simulink model "Model_3_1"  (R2021a)
settings: Solver=VariableStepAuto  StartTime=0.0  StopTime=10  RelTol=1e-3
InitFcn:
  | bx=0; %25
  | bl=0; %50
  | bc=0.01;
  | 
  | ml=2; %2
  | 
  | mc=0.5;
  | M2=0.5;
  | 
  | mt=5;
  | g=9.81;
  | l_ref=0.1;
  | l_ini=1;
  | l=l_ini;
  | x_ref=1; %5 3
  | n1=1; %5
  | n2=1;
  | 
  | L_2=0;  %chieu dai day nang ha
  | 
  | theta1_ini=0*pi/180;
  | theta2_ini=0*pi/180;  %2*pi/180
  | 
  | L_tai=0.2;
  | %ADRC' s parameter caculation
  | %b0 = (1)/(mc+mt+ml);
  | b0=(ml+mc)/(mt*mc+2*ml*mc+mt*ml+ml^2+mc^2); %Enhanced-coupling
  | %k_ESO = 100;
  | k_ESO = 100;
  | T_set  = 3; %5; 3
  | 
  | s_cl = -5.85/T_set;
  | Kp   = s_cl^2;
  | Kd   = -2*s_cl;
  | 
  | s_ESO = k_ESO*s_cl;
  | l1        = -3*s_ESO;
  | l2        = 3*( s_ESO)^2;
  | l3        = -(s_ESO)^3;
  | 
  | %b1 = (mt+mc)/(mc*ml +mc*mt+ml*mt);
  | b1=1/(ml+mc);
  | k_ESO1 =100; %100
  | T_set1  = 3;   %3
  | s_cl1 = -5.85/T_set1;
  | Kp1   = s_cl1^2;
  | Kd1   = -2*s_cl1;
  | 
  | s_ESO1 = k_ESO1*s_cl1;
  | l11        = -3*s_ESO1;
  | l21        = 3*( s_ESO1)^2;
  | l31        = -(s_ESO1)^3;
  | 
  | 
  | %L1=l_ini;
  | L11=0.55;
  | L2=0.1;
  | m1=2;
  | %m2=M2;
  | m=5;
  | ... (+39 lines)
libraries: neural x1137, simulink x36, simulink_extras x4
(part 6 of 45)

== system Model_3_1/26_12_theta1 bang 0 n1=5; n2=1 /Subsystem1/Fitness APS 1 ==
  e : Inport
  Abs : Abs
  Abs1 : Abs
  Integrator : Integrator
  MinMax Running Resettable : simulink/Math Operations/MinMax Running Resettable  Function=max  vinit=0.0
  Step : Step  Time=0.000001  Before=1  After=0  SampleTime=0
  IAE : Outport
  MAx : Outport  Port=2
  wires:
  Abs/1 -> Integrator/1
  Abs1/1 -> MinMax Running Resettable/1
  Step/1 -> MinMax Running Resettable/2
  e/1 -> Abs/1, Abs1/1
  Integrator/1 -> IAE/1
  MinMax Running Resettable/1 -> MAx/1

== system Model_3_1/26_12_theta1 bang 0 n1=5; n2=1 /Subsystem1/Fitness APS 2 ==
  e : Inport
  Abs : Abs
  Abs1 : Abs
  Integrator : Integrator
  MinMax Running Resettable : simulink/Math Operations/MinMax Running Resettable  Function=max  vinit=0.0
  Step : Step  Time=0.000001  Before=1  After=0  SampleTime=0
  IAE : Outport
  MAx : Outport  Port=2
  wires:
  Abs/1 -> Integrator/1
  Abs1/1 -> MinMax Running Resettable/1
  Step/1 -> MinMax Running Resettable/2
  e/1 -> Abs/1, Abs1/1
  Integrator/1 -> IAE/1
  MinMax Running Resettable/1 -> MAx/1

== system Model_3_1/26_12_theta1 bang 0 n1=5; n2=1 /Subsystem2/Fitness APS 1 ==
  e : Inport
  Abs : Abs
  Abs1 : Abs
  Integrator : Integrator
  MinMax Running Resettable : simulink/Math Operations/MinMax Running Resettable  Function=max  vinit=0.0
  Step : Step  Time=0.000001  Before=1  After=0  SampleTime=0
  IAE : Outport
  MAx : Outport  Port=2
  wires:
  Abs/1 -> Integrator/1
  Abs1/1 -> MinMax Running Resettable/1
  Step/1 -> MinMax Running Resettable/2
  e/1 -> Abs/1, Abs1/1
  Integrator/1 -> IAE/1
  MinMax Running Resettable/1 -> MAx/1

== system Model_3_1/26_12_theta1 bang 0 n1=5; n2=1 /Subsystem2/Fitness APS 2 ==
  e : Inport
  Abs : Abs
  Abs1 : Abs
  Integrator : Integrator
  MinMax Running Resettable : simulink/Math Operations/MinMax Running Resettable  Function=max  vinit=0.0
  Step : Step  Time=0.000001  Before=1  After=0  SampleTime=0
  IAE : Outport
  MAx : Outport  Port=2
  wires:
  Abs/1 -> Integrator/1
  Abs1/1 -> MinMax Running Resettable/1
  Step/1 -> MinMax Running Resettable/2
  e/1 -> Abs/1, Abs1/1
  Integrator/1 -> IAE/1
  MinMax Running Resettable/1 -> MAx/1

== system Model_3_1/26_12_theta1 bang 0 n1=5; n2=1 /Subsystem3/Fitness APS 1 ==
  e : Inport
  Abs : Abs
  Abs1 : Abs
  Integrator : Integrator
  MinMax Running Resettable : simulink/Math Operations/MinMax Running Resettable  Function=max  vinit=0.0
  Step : Step  Time=0.000001  Before=1  After=0  SampleTime=0
  IAE : Outport
  MAx : Outport  Port=2
  wires:
  Abs/1 -> Integrator/1
  Abs1/1 -> MinMax Running Resettable/1
  Step/1 -> MinMax Running Resettable/2
  e/1 -> Abs/1, Abs1/1
  Integrator/1 -> IAE/1
  MinMax Running Resettable/1 -> MAx/1

== system Model_3_1/26_12_theta1 bang 0 n1=5; n2=1 /Subsystem3/Fitness APS 2 ==
  e : Inport
  Abs : Abs
  Abs1 : Abs
  Integrator : Integrator
  MinMax Running Resettable : simulink/Math Operations/MinMax Running Resettable  Function=max  vinit=0.0
  Step : Step  Time=0.000001  Before=1  After=0  SampleTime=0
  IAE : Outport
  MAx : Outport  Port=2
  wires:
  Abs/1 -> Integrator/1
  Abs1/1 -> MinMax Running Resettable/1
  Step/1 -> MinMax Running Resettable/2
  e/1 -> Abs/1, Abs1/1
  Integrator/1 -> IAE/1
  MinMax Running Resettable/1 -> MAx/1

== system Model_3_1/26_12_theta1 bang 0 n1=5; n2=1 /Subsystem4/Fitness APS 1 ==
  e : Inport
  Abs : Abs
  Abs1 : Abs
  Integrator : Integrator
  MinMax Running Resettable : simulink/Math Operations/MinMax Running Resettable  Function=max  vinit=0.0
  Step : Step  Time=0.000001  Before=1  After=0  SampleTime=0
  IAE : Outport
  MAx : Outport  Port=2
  wires:
  Abs/1 -> Integrator/1
  Abs1/1 -> MinMax Running Resettable/1
  Step/1 -> MinMax Running Resettable/2
  e/1 -> Abs/1, Abs1/1
  Integrator/1 -> IAE/1
  MinMax Running Resettable/1 -> MAx/1

== system Model_3_1/26_12_theta1 bang 0 n1=5; n2=1 /Subsystem4/Fitness APS 2 ==
  e : Inport
  Abs : Abs
  Abs1 : Abs
  Integrator : Integrator
  MinMax Running Resettable : simulink/Math Operations/MinMax Running Resettable  Function=max  vinit=0.0
  Step : Step  Time=0.000001  Before=1  After=0  SampleTime=0
  IAE : Outport
  MAx : Outport  Port=2
  wires:
  Abs/1 -> Integrator/1
  Abs1/1 -> MinMax Running Resettable/1
  Step/1 -> MinMax Running Resettable/2
  e/1 -> Abs/1, Abs1/1
  Integrator/1 -> IAE/1
  MinMax Running Resettable/1 -> MAx/1

== system Model_3_1/26_12_theta1 bang 0 n1=5; n2=1 /Subsystem5/Fitness APS 1 ==
  e : Inport
  Abs : Abs
  Abs1 : Abs
  Integrator : Integrator
  MinMax Running Resettable : simulink/Math Operations/MinMax Running Resettable  Function=max  vinit=0.0
  Step : Step  Time=0.000001  Before=1  After=0  SampleTime=0
  IAE : Outport
  MAx : Outport  Port=2
  wires:
  Abs/1 -> Integrator/1
  Abs1/1 -> MinMax Running Resettable/1
  Step/1 -> MinMax Running Resettable/2
  e/1 -> Abs/1, Abs1/1
  Integrator/1 -> IAE/1
  MinMax Running Resettable/1 -> MAx/1

== system Model_3_1/26_12_theta1 bang 0 n1=5; n2=1 /Subsystem5/Fitness APS 2 ==
  e : Inport
  Abs : Abs
  Abs1 : Abs
  Integrator : Integrator
  MinMax Running Resettable : simulink/Math Operations/MinMax Running Resettable  Function=max  vinit=0.0
  Step : Step  Time=0.000001  Before=1  After=0  SampleTime=0
  IAE : Outport
  MAx : Outport  Port=2
  wires:
  Abs/1 -> Integrator/1
  Abs1/1 -> MinMax Running Resettable/1
  Step/1 -> MinMax Running Resettable/2
  e/1 -> Abs/1, Abs1/1
  Integrator/1 -> IAE/1
  MinMax Running Resettable/1 -> MAx/1

== system Model_3_1/26_12_theta1 bang 0 n1=5; n2=1 /Subsystem6/Fitness APS 1 ==
  e : Inport
  Abs : Abs
  Abs1 : Abs
  Integrator : Integrator
  MinMax Running Resettable : simulink/Math Operations/MinMax Running Resettable  Function=max  vinit=0.0
  Step : Step  Time=0.000001  Before=1  After=0  SampleTime=0
  IAE : Outport
  MAx : Outport  Port=2
  wires:
  Abs/1 -> Integrator/1
  Abs1/1 -> MinMax Running Resettable/1
  Step/1 -> MinMax Running Resettable/2
  e/1 -> Abs/1, Abs1/1
  Integrator/1 -> IAE/1
  MinMax Running Resettable/1 -> MAx/1

== system Model_3_1/26_12_theta1 bang 0 n1=5; n2=1 /Subsystem6/Fitness APS 2 ==
  e : Inport
  Abs : Abs
  Abs1 : Abs
  Integrator : Integrator
  MinMax Running Resettable : simulink/Math Operations/MinMax Running Resettable  Function=max  vinit=0.0
  Step : Step  Time=0.000001  Before=1  After=0  SampleTime=0
  IAE : Outport
  MAx : Outport  Port=2
  wires:
  Abs/1 -> Integrator/1
  Abs1/1 -> MinMax Running Resettable/1
  Step/1 -> MinMax Running Resettable/2
  e/1 -> Abs/1, Abs1/1
  Integrator/1 -> IAE/1
  MinMax Running Resettable/1 -> MAx/1

== system Model_3_1/26_12_theta1 bang 0 n1=5; n2=1 /ko co FL_25.12_2/Layer 1 ==
  "p{1}" : Inport  PortDimensions=2
      mask Display: e = 0.06;c1 = [120 230 180]/255;c2 = ([120 230 180]+0)/(256+128);c3 = ([120 230 180]+128)/(256+128);patch([0 1 1 0],[0 0 1 1],c1);patch([0 1 1 1-e 1-e 0+e],[0 0 1 1-e 0+e 0+e],c2);patch([0 0 1 1-e 0+e 0+e],[0 1 1 1-e 1-e 0+e],c3);plot([0 1 1 0 0],[0 0 1 1 0]);
  Delays 1 : Subsystem
      mask Display: e = 0.06;c1 = [120 150 230]/255;c2 = ([120 150 230]+0)/383;c3 = ([120 150 230]+128)/383;patch([0 1 1 0],[0 0 1 1],c1);patch([0 1 1 1-e 1-e 0+e],[0 0 1 1-e 0+e 0+e],c2);patch([0 0 1 1-e 0+e 0+e],[0 1 1 1-e 1-e 0+e],c3);plot([0 1 1 0 0],[0 0 1 1 0]);disp('0');
  "IW{1,1}" : Subsystem
      mask Display: e = 0.06;c1 = [120 150 230]/255;c2 = ([120 150 230]+0)/383;c3 = ([120 150 230]+128)/383;patch([0 1 1 0],[0 0 1 1],c1);patch([0 1 1 1-e 1-e 0+e],[0 0 1 1-e 0+e 0+e],c2);patch([0 0 1 1-e 0+e 0+e],[0 1 1 1-e 1-e 0+e],c3);plot([0 1 1 0 0],[0 0 1 1 0]);disp('W');
  "b{1}" : Constant  Value=[0.83255461115769768820626950400765053927898406982421875;0.83255461115769768820626950400765053927898406982421875;0.83255461115769768820626950400765053927898406982421875;0.83255461115769768820626950400765053927898406982421875;0.83255461115769768820626950400765053927898406982421875;0.83255461115769768820626950400765053927898406982421875;0.83255461115769768820626950400765053927898406982421875;0.83255461115769768820626950400765053927898406982421875;0.83255461115769768820626950400765053927898406982421875;0.83255461115769768820626950400765053927898406982421875;0.83255461115769768820626950400765053927898406982421875;0.83255461115769768820626950400765053927898406982421875;0.83255461115769768820626950400765053927898406982421875;0.83255461115769768820626950400765053927898406982421875;0.83255461115769768820626950400765053927898406982421875;0.83255461115769768820626950400765053927898406982421875;0.83255461115769768820626950400765053927898406982421875;0.83255461115769768820626950400765053927898406982421875;0.83255461115769768820626950400765053927898406982421875;0.83255461115769768820626950400765053927898406982421875;0.83255461115769768820626950400765053927898406982421875;0.83255461115769768820626950400765053927898406982421875;0.83255461115769768820626950400765053927898406982421875;0.83255461115769768820626950400765053927898406982421875;0.83255461115769768820626950400765053927898406982421875;0.83255461115769768820626950400765053927898406982421875;0.83255461115769768820626950400765053927898406982421875;0.83255461115769768820626950400765053927898406982421875;0.83255461115769768820626950400765053927898406982421875;0.83255461115769768820626950400765053927898406982421875;0.83255461115769768820626950400765053927898406982421875;0.83255461115769768820626950400765053927898406982421875;0.83255461115769768820626950400765053927898406982421875;0.83255461115769768820626950400765053927898406982421875;0.83255461115769768820626950400765053927898406982421875;0.83255461115769768820626950400765053927898406982421875;0.83255461115769768820626950400765053927898406982421875;0.83255461115769768820626950400765053927898406982421875;0.83255461115769768820626950400765053927898406982421875;0.83255461115769768820626950400765053927898406982421875;0.83255461115769768820626950400765053927898406982421875;0.83255461115769768820626950400765053927898406982421875;0.83255461115769768820626950400765053927898406982421875;0.83255461115769768820626950400765053927898406982421875;0.83255461115769768820626950400765053927898406982421875;0.83255461115769768820626950400765053927898406982421875]
      mask Display: e = 0.06;c1 = [120 150 230]/255;c2 = ([120 150 230]+0)/383;c3 = ([120 150 230]+128)/383;patch([0 1 1 0],[0 0 1 1],c1);patch([0 1 1 1-e 1-e 0+e],[0 0 1 1-e 0+e 0+e],c2);patch([0 0 1 1-e 0+e 0+e],[0 1 1 1-e 1-e 0+e],c3);plot([0 1 1 0 0],[0 0 1 1 0]);disp('b');
  netprod : Product  InputSameDT=on  RndMeth=Zero  SaturateOnIntegerOverflow=on  OutDataTypeStr=Inherit: Same as first input
      mask Display: e = 0.06;c1 = [120 150 230]/255;c2 = ([120 150 230]+0)/383;c3 = ([120 150 230]+128)/383;patch([0 1 1 0],[0 0 1 1],c1);patch([0 1 1 1-e 1-e 0+e],[0 0 1 1-e 0+e 0+e],c2);patch([0 0 1 1-e 0+e 0+e],[0 1 1 1-e 1-e 0+e],c3);plot([0 1 1 0 0],[0 0 1 1 0]);disp('*');
  radbas : neural/Transfer Functions/radbas
      settings: SourceProductBaseCode=NN
  "a{1}" : Outport  InitialOutput=[0;0;0;0;0;0;0;0;0;0;0;0;0;0;0;0;0;0;0;0;0;0;0;0;0;0;0;0;0;0;0;0;0;0;0;0;0;0;0;0;0;0;0;0;0;0]
      mask Display: e = 0.06;c1 = [120 230 180]/255;c2 = ([120 230 180]+0)/(256+128);c3 = ([120 230 180]+128)/(256+128);patch([0 1 1 0],[0 0 1 1],c1);patch([0 1 1 1-e 1-e 0+e],[0 0 1 1-e 0+e 0+e],c2);patch([0 0 1 1-e 0+e 0+e],[0 1 1 1-e 1-e 0+e],c3);plot([0 1 1 0 0],[0 0 1 1 0]);
  wires:
  "p{1}"/1 -> Delays 1/1("p{1}")
  Delays 1/1("pd{1,1}") -> "IW{1,1}"/1("pd{1,1}")
  "IW{1,1}"/1("iz{1,1}") -> netprod/1
  "b{1}"/1 -> netprod/2
  netprod/1 -> radbas/1
  radbas/1 -> "a{1}"/1

== system Model_3_1/26_12_theta1 bang 0 n1=5; n2=1 /ko co FL_25.12_2/Layer 2 ==
  "a{1} " : Inport  PortDimensions=46
      mask Display: e = 0.06;c1 = [120 230 180]/255;c2 = ([120 230 180]+0)/(256+128);c3 = ([120 230 180]+128)/(256+128);patch([0 1 1 0],[0 0 1 1],c1);patch([0 1 1 1-e 1-e 0+e],[0 0 1 1-e 0+e 0+e],c2);patch([0 0 1 1-e 0+e 0+e],[0 1 1 1-e 1-e 0+e],c3);plot([0 1 1 0 0],[0 0 1 1 0]);
  Delays 1 : Subsystem
      mask Display: e = 0.06;c1 = [120 150 230]/255;c2 = ([120 150 230]+0)/383;c3 = ([120 150 230]+128)/383;patch([0 1 1 0],[0 0 1 1],c1);patch([0 1 1 1-e 1-e 0+e],[0 0 1 1-e 0+e 0+e],c2);patch([0 0 1 1-e 0+e 0+e],[0 1 1 1-e 1-e 0+e],c3);plot([0 1 1 0 0],[0 0 1 1 0]);disp('0');
  "LW{2,1}" : Subsystem
      mask Display: e = 0.06;c1 = [120 150 230]/255;c2 = ([120 150 230]+0)/383;c3 = ([120 150 230]+128)/383;patch([0 1 1 0],[0 0 1 1],c1);patch([0 1 1 1-e 1-e 0+e],[0 0 1 1-e 0+e 0+e],c2);patch([0 0 1 1-e 0+e 0+e],[0 1 1 1-e 1-e 0+e],c3);plot([0 1 1 0 0],[0 0 1 1 0]);disp('W');
  "b{2}" : Constant  Value=[-128346.528805981113691814243793487548828125;1328.286650372559279276174493134021759033203125;-25277.92810932771317311562597751617431640625]
      mask Display: e = 0.06;c1 = [120 150 230]/255;c2 = ([120 150 230]+0)/383;c3 = ([120 150 230]+128)/383;patch([0 1 1 0],[0 0 1 1],c1);patch([0 1 1 1-e 1-e 0+e],[0 0 1 1-e 0+e 0+e],c2);patch([0 0 1 1-e 0+e 0+e],[0 1 1 1-e 1-e 0+e],c3);plot([0 1 1 0 0],[0 0 1 1 0]);disp('b');
  netsum : Sum  Inputs=2  InputSameDT=on  SaturateOnIntegerOverflow=on  OutDataTypeStr=Inherit: Same as first input
      mask Display: e = 0.06;c1 = [120 150 230]/255;c2 = ([120 150 230]+0)/383;c3 = ([120 150 230]+128)/383;patch([0 1 1 0],[0 0 1 1],c1);patch([0 1 1 1-e 1-e 0+e],[0 0 1 1-e 0+e 0+e],c2);patch([0 0 1 1-e 0+e 0+e],[0 1 1 1-e 1-e 0+e],c3);plot([0 1 1 0 0],[0 0 1 1 0]);disp('+');
  purelin : neural/Transfer Functions/purelin
  "a{2}" : Outport  InitialOutput=[0;0;0]
      mask Display: e = 0.06;c1 = [120 230 180]/255;c2 = ([120 230 180]+0)/(256+128);c3 = ([120 230 180]+128)/(256+128);patch([0 1 1 0],[0 0 1 1],c1);patch([0 1 1 1-e 1-e 0+e],[0 0 1 1-e 0+e 0+e],c2);patch([0 0 1 1-e 0+e 0+e],[0 1 1 1-e 1-e 0+e],c3);plot([0 1 1 0 0],[0 0 1 1 0]);
  wires:
  "a{1} "/1 -> Delays 1/1("p{2}")
  Delays 1/1("pd{2,1}") -> "LW{2,1}"/1("ad{2,1}")
  "LW{2,1}"/1("lz{2,1}") -> netsum/1
  "b{2}"/1 -> netsum/2
  netsum/1 -> purelin/1
  purelin/1 -> "a{2}"/1

== system Model_3_1/26_12_theta1 bang 0 n1=5; n2=1 /ko co FL_25.12_2/Process Input 1 ==
  x : Inport  PortDimensions=2
      mask Display: e = 0.06;c1 = [120 230 180]/255;c2 = ([120 230 180]+0)/(256+128);c3 = ([120 230 180]+128)/(256+128);patch([0 1 1 0],[0 0 1 1],c1);patch([0 1 1 1-e 1-e 0+e],[0 0 1 1-e 0+e 0+e],c2);patch([0 0 1 1-e 0+e 0+e],[0 1 1 1-e 1-e 0+e],c3);plot([0 1 1 0 0],[0 0 1 1 0]);
  p : Outport  PortDimensions=2
      mask Display: e = 0.06;c1 = [120 230 180]/255;c2 = ([120 230 180]+0)/(256+128);c3 = ([120 230 180]+128)/(256+128);patch([0 1 1 0],[0 0 1 1],c1);patch([0 1 1 1-e 1-e 0+e],[0 0 1 1-e 0+e 0+e],c2);patch([0 0 1 1-e 0+e 0+e],[0 1 1 1-e 1-e 0+e],c3);plot([0 1 1 0 0],[0 0 1 1 0]);
  wires:
  x/1 -> p/1

== system Model_3_1/26_12_theta1 bang 0 n1=5; n2=1 /ko co FL_25.12_2/Process Output 1 ==
  a : Inport  PortDimensions=3
      mask Display: e = 0.06;c1 = [120 230 180]/255;c2 = ([120 230 180]+0)/(256+128);c3 = ([120 230 180]+128)/(256+128);patch([0 1 1 0],[0 0 1 1],c1);patch([0 1 1 1-e 1-e 0+e],[0 0 1 1-e 0+e 0+e],c2);patch([0 0 1 1-e 0+e 0+e],[0 1 1 1-e 1-e 0+e],c3);plot([0 1 1 0 0],[0 0 1 1 0]);
  y : Outport  PortDimensions=3
      mask Display: e = 0.06;c1 = [120 230 180]/255;c2 = ([120 230 180]+0)/(256+128);c3 = ([120 230 180]+128)/(256+128);patch([0 1 1 0],[0 0 1 1],c1);patch([0 1 1 1-e 1-e 0+e],[0 0 1 1-e 0+e 0+e],c2);patch([0 0 1 1-e 0+e 0+e],[0 1 1 1-e 1-e 0+e],c3);plot([0 1 1 0 0],[0 0 1 1 0]);
  wires:
  a/1 -> y/1

== system Model_3_1/26_12_theta1 bang 0 n1=5; n2=1 /ko co FL_26.1_1/Layer 1 ==
  "p{1}" : Inport  PortDimensions=2
      mask Display: e = 0.06;c1 = [120 230 180]/255;c2 = ([120 230 180]+0)/(256+128);c3 = ([120 230 180]+128)/(256+128);patch([0 1 1 0],[0 0 1 1],c1);patch([0 1 1 1-e 1-e 0+e],[0 0 1 1-e 0+e 0+e],c2);patch([0 0 1 1-e 0+e 0+e],[0 1 1 1-e 1-e 0+e],c3);plot([0 1 1 0 0],[0 0 1 1 0]);
  Delays 1 : Subsystem
      mask Display: e = 0.06;c1 = [120 150 230]/255;c2 = ([120 150 230]+0)/383;c3 = ([120 150 230]+128)/383;patch([0 1 1 0],[0 0 1 1],c1);patch([0 1 1 1-e 1-e 0+e],[0 0 1 1-e 0+e 0+e],c2);patch([0 0 1 1-e 0+e 0+e],[0 1 1 1-e 1-e 0+e],c3);plot([0 1 1 0 0],[0 0 1 1 0]);disp('0');
  "IW{1,1}" : Subsystem
      mask Display: e = 0.06;c1 = [120 150 230]/255;c2 = ([120 150 230]+0)/383;c3 = ([120 150 230]+128)/383;patch([0 1 1 0],[0 0 1 1],c1);patch([0 1 1 1-e 1-e 0+e],[0 0 1 1-e 0+e 0+e],c2);patch([0 0 1 1-e 0+e 0+e],[0 1 1 1-e 1-e 0+e],c3);plot([0 1 1 0 0],[0 0 1 1 0]);disp('W');
  "b{1}" : Constant  Value=[0.83255461115769768820626950400765053927898406982421875;0.83255461115769768820626950400765053927898406982421875;0.83255461115769768820626950400765053927898406982421875;0.83255461115769768820626950400765053927898406982421875;0.83255461115769768820626950400765053927898406982421875;0.83255461115769768820626950400765053927898406982421875;0.83255461115769768820626950400765053927898406982421875;0.83255461115769768820626950400765053927898406982421875;0.83255461115769768820626950400765053927898406982421875;0.83255461115769768820626950400765053927898406982421875;0.83255461115769768820626950400765053927898406982421875;0.83255461115769768820626950400765053927898406982421875;0.83255461115769768820626950400765053927898406982421875;0.83255461115769768820626950400765053927898406982421875;0.83255461115769768820626950400765053927898406982421875;0.83255461115769768820626950400765053927898406982421875;0.83255461115769768820626950400765053927898406982421875;0.83255461115769768820626950400765053927898406982421875;0.83255461115769768820626950400765053927898406982421875;0.83255461115769768820626950400765053927898406982421875;0.83255461115769768820626950400765053927898406982421875;0.83255461115769768820626950400765053927898406982421875;0.83255461115769768820626950400765053927898406982421875;0.83255461115769768820626950400765053927898406982421875;0.83255461115769768820626950400765053927898406982421875;0.83255461115769768820626950400765053927898406982421875;0.83255461115769768820626950400765053927898406982421875;0.83255461115769768820626950400765053927898406982421875;0.83255461115769768820626950400765053927898406982421875;0.83255461115769768820626950400765053927898406982421875;0.83255461115769768820626950400765053927898406982421875;0.83255461115769768820626950400765053927898406982421875;0.83255461115769768820626950400765053927898406982421875;0.83255461115769768820626950400765053927898406982421875;0.83255461115769768820626950400765053927898406982421875;0.83255461115769768820626950400765053927898406982421875;0.83255461115769768820626950400765053927898406982421875;0.83255461115769768820626950400765053927898406982421875;0.83255461115769768820626950400765053927898406982421875;0.83255461115769768820626950400765053927898406982421875;0.83255461115769768820626950400765053927898406982421875;0.83255461115769768820626950400765053927898406982421875;0.83255461115769768820626950400765053927898406982421875;0.83255461115769768820626950400765053927898406982421875;0.83255461115769768820626950400765053927898406982421875;0.83255461115769768820626950400765053927898406982421875]
      mask Display: e = 0.06;c1 = [120 150 230]/255;c2 = ([120 150 230]+0)/383;c3 = ([120 150 230]+128)/383;patch([0 1 1 0],[0 0 1 1],c1);patch([0 1 1 1-e 1-e 0+e],[0 0 1 1-e 0+e 0+e],c2);patch([0 0 1 1-e 0+e 0+e],[0 1 1 1-e 1-e 0+e],c3);plot([0 1 1 0 0],[0 0 1 1 0]);disp('b');
  netprod : Product  InputSameDT=on  RndMeth=Zero  SaturateOnIntegerOverflow=on  OutDataTypeStr=Inherit: Same as first input
      mask Display: e = 0.06;c1 = [120 150 230]/255;c2 = ([120 150 230]+0)/383;c3 = ([120 150 230]+128)/383;patch([0 1 1 0],[0 0 1 1],c1);patch([0 1 1 1-e 1-e 0+e],[0 0 1 1-e 0+e 0+e],c2);patch([0 0 1 1-e 0+e 0+e],[0 1 1 1-e 1-e 0+e],c3);plot([0 1 1 0 0],[0 0 1 1 0]);disp('*');
  radbas : neural/Transfer Functions/radbas
      settings: SourceProductBaseCode=NN
  "a{1}" : Outport  InitialOutput=[0;0;0;0;0;0;0;0;0;0;0;0;0;0;0;0;0;0;0;0;0;0;0;0;0;0;0;0;0;0;0;0;0;0;0;0;0;0;0;0;0;0;0;0;0;0]
      mask Display: e = 0.06;c1 = [120 230 180]/255;c2 = ([120 230 180]+0)/(256+128);c3 = ([120 230 180]+128)/(256+128);patch([0 1 1 0],[0 0 1 1],c1);patch([0 1 1 1-e 1-e 0+e],[0 0 1 1-e 0+e 0+e],c2);patch([0 0 1 1-e 0+e 0+e],[0 1 1 1-e 1-e 0+e],c3);plot([0 1 1 0 0],[0 0 1 1 0]);
  wires:
  "p{1}"/1 -> Delays 1/1("p{1}")
  Delays 1/1("pd{1,1}") -> "IW{1,1}"/1("pd{1,1}")
  "IW{1,1}"/1("iz{1,1}") -> netprod/1
  "b{1}"/1 -> netprod/2
  netprod/1 -> radbas/1
  radbas/1 -> "a{1}"/1

== system Model_3_1/26_12_theta1 bang 0 n1=5; n2=1 /ko co FL_26.1_1/Layer 2 ==
  "a{1} " : Inport  PortDimensions=46
      mask Display: e = 0.06;c1 = [120 230 180]/255;c2 = ([120 230 180]+0)/(256+128);c3 = ([120 230 180]+128)/(256+128);patch([0 1 1 0],[0 0 1 1],c1);patch([0 1 1 1-e 1-e 0+e],[0 0 1 1-e 0+e 0+e],c2);patch([0 0 1 1-e 0+e 0+e],[0 1 1 1-e 1-e 0+e],c3);plot([0 1 1 0 0],[0 0 1 1 0]);
  Delays 1 : Subsystem
      mask Display: e = 0.06;c1 = [120 150 230]/255;c2 = ([120 150 230]+0)/383;c3 = ([120 150 230]+128)/383;patch([0 1 1 0],[0 0 1 1],c1);patch([0 1 1 1-e 1-e 0+e],[0 0 1 1-e 0+e 0+e],c2);patch([0 0 1 1-e 0+e 0+e],[0 1 1 1-e 1-e 0+e],c3);plot([0 1 1 0 0],[0 0 1 1 0]);disp('0');
  "LW{2,1}" : Subsystem
      mask Display: e = 0.06;c1 = [120 150 230]/255;c2 = ([120 150 230]+0)/383;c3 = ([120 150 230]+128)/383;patch([0 1 1 0],[0 0 1 1],c1);patch([0 1 1 1-e 1-e 0+e],[0 0 1 1-e 0+e 0+e],c2);patch([0 0 1 1-e 0+e 0+e],[0 1 1 1-e 1-e 0+e],c3);plot([0 1 1 0 0],[0 0 1 1 0]);disp('W');
  "b{2}" : Constant  Value=[-121700.422889903260511346161365509033203125;2285.68691207953406774322502315044403076171875;-58069.0026805897723534144461154937744140625]
      mask Display: e = 0.06;c1 = [120 150 230]/255;c2 = ([120 150 230]+0)/383;c3 = ([120 150 230]+128)/383;patch([0 1 1 0],[0 0 1 1],c1);patch([0 1 1 1-e 1-e 0+e],[0 0 1 1-e 0+e 0+e],c2);patch([0 0 1 1-e 0+e 0+e],[0 1 1 1-e 1-e 0+e],c3);plot([0 1 1 0 0],[0 0 1 1 0]);disp('b');
  netsum : Sum  Inputs=2  InputSameDT=on  SaturateOnIntegerOverflow=on  OutDataTypeStr=Inherit: Same as first input
      mask Display: e = 0.06;c1 = [120 150 230]/255;c2 = ([120 150 230]+0)/383;c3 = ([120 150 230]+128)/383;patch([0 1 1 0],[0 0 1 1],c1);patch([0 1 1 1-e 1-e 0+e],[0 0 1 1-e 0+e 0+e],c2);patch([0 0 1 1-e 0+e 0+e],[0 1 1 1-e 1-e 0+e],c3);plot([0 1 1 0 0],[0 0 1 1 0]);disp('+');
  purelin : neural/Transfer Functions/purelin
  "a{2}" : Outport  InitialOutput=[0;0;0]
      mask Display: e = 0.06;c1 = [120 230 180]/255;c2 = ([120 230 180]+0)/(256+128);c3 = ([120 230 180]+128)/(256+128);patch([0 1 1 0],[0 0 1 1],c1);patch([0 1 1 1-e 1-e 0+e],[0 0 1 1-e 0+e 0+e],c2);patch([0 0 1 1-e 0+e 0+e],[0 1 1 1-e 1-e 0+e],c3);plot([0 1 1 0 0],[0 0 1 1 0]);
  wires:
  "a{1} "/1 -> Delays 1/1("p{2}")
  Delays 1/1("pd{2,1}") -> "LW{2,1}"/1("ad{2,1}")
  "LW{2,1}"/1("lz{2,1}") -> netsum/1
  "b{2}"/1 -> netsum/2
  netsum/1 -> purelin/1
  purelin/1 -> "a{2}"/1

== system Model_3_1/26_12_theta1 bang 0 n1=5; n2=1 /ko co FL_26.1_1/Process Input 1 ==
  x : Inport  PortDimensions=2
      mask Display: e = 0.06;c1 = [120 230 180]/255;c2 = ([120 230 180]+0)/(256+128);c3 = ([120 230 180]+128)/(256+128);patch([0 1 1 0],[0 0 1 1],c1);patch([0 1 1 1-e 1-e 0+e],[0 0 1 1-e 0+e 0+e],c2);patch([0 0 1 1-e 0+e 0+e],[0 1 1 1-e 1-e 0+e],c3);plot([0 1 1 0 0],[0 0 1 1 0]);
  p : Outport  PortDimensions=2
      mask Display: e = 0.06;c1 = [120 230 180]/255;c2 = ([120 230 180]+0)/(256+128);c3 = ([120 230 180]+128)/(256+128);patch([0 1 1 0],[0 0 1 1],c1);patch([0 1 1 1-e 1-e 0+e],[0 0 1 1-e 0+e 0+e],c2);patch([0 0 1 1-e 0+e 0+e],[0 1 1 1-e 1-e 0+e],c3);plot([0 1 1 0 0],[0 0 1 1 0]);
  wires:
  x/1 -> p/1

== system Model_3_1/26_12_theta1 bang 0 n1=5; n2=1 /ko co FL_26.1_1/Process Output 1 ==
  a : Inport  PortDimensions=3
      mask Display: e = 0.06;c1 = [120 230 180]/255;c2 = ([120 230 180]+0)/(256+128);c3 = ([120 230 180]+128)/(256+128);patch([0 1 1 0],[0 0 1 1],c1);patch([0 1 1 1-e 1-e 0+e],[0 0 1 1-e 0+e 0+e],c2);patch([0 0 1 1-e 0+e 0+e],[0 1 1 1-e 1-e 0+e],c3);plot([0 1 1 0 0],[0 0 1 1 0]);
  y : Outport  PortDimensions=3
      mask Display: e = 0.06;c1 = [120 230 180]/255;c2 = ([120 230 180]+0)/(256+128);c3 = ([120 230 180]+128)/(256+128);patch([0 1 1 0],[0 0 1 1],c1);patch([0 1 1 1-e 1-e 0+e],[0 0 1 1-e 0+e 0+e],c2);patch([0 0 1 1-e 0+e 0+e],[0 1 1 1-e 1-e 0+e],c3);plot([0 1 1 0 0],[0 0 1 1 0]);
  wires:
  a/1 -> y/1

== system Model_3_1/3_1_theta1 bang 0 n1=1; n2=1 2/ETM1/ETM1 ==
  In1 : Inport
  Gain : Gain  Gain=A1_etm4_1
  Gain1 : Gain  Gain=A2_etm4_1
  Gain2 : Gain  Gain=A3_etm4_1
  Gain3 : Gain  Gain=A4_etm4_1
  Sum : Sum  Inputs=++++
  Transport Delay : TransportDelay  DelayTime=t1_etm4_1
  Transport Delay1 : TransportDelay  DelayTime=t2_etm4_1
  Transport Delay2 : TransportDelay  DelayTime=t3_etm4_1
  Out1 : Outport
  wires:
  In1/1 -> Gain1/1, Gain3/1, Gain2/1, Gain/1
  Gain1/1 -> Transport Delay/1
  Transport Delay/1 -> Sum/2
  Sum/1 -> Out1/1
  Gain2/1 -> Transport Delay1/1
  Gain/1 -> Sum/1
  Transport Delay1/1 -> Sum/3
  Gain3/1 -> Transport Delay2/1
  Transport Delay2/1 -> Sum/4

== system Model_3_1/3_1_theta1 bang 0 n1=1; n2=1 2/ETM1/ETM4 ==
  In1 : Inport
  Gain : Gain  Gain=A1_etm4_2
  Gain1 : Gain  Gain=A2_etm4_2
  Gain2 : Gain  Gain=A3_etm4_2
  Gain3 : Gain  Gain=A4_etm4_2
  Sum : Sum  Inputs=++++
  Transport Delay : TransportDelay  DelayTime=t1_etm4_2
  Transport Delay1 : TransportDelay  DelayTime=t2_etm4_2
  Transport Delay2 : TransportDelay  DelayTime=t3_etm4_2
  Out1 : Outport
  wires:
  In1/1 -> Gain1/1, Gain3/1, Gain2/1, Gain/1
  Gain1/1 -> Transport Delay/1
  Transport Delay/1 -> Sum/2
  Sum/1 -> Out1/1
  Gain2/1 -> Transport Delay1/1
  Gain/1 -> Sum/1
  Transport Delay1/1 -> Sum/3
  Gain3/1 -> Transport Delay2/1
  Transport Delay2/1 -> Sum/4

== system Model_3_1/3_1_theta1 bang 0 n1=1; n2=1 2/ETM2/ETM1 ==
  In1 : Inport
  Gain : Gain  Gain=A1_etm4_1
  Gain1 : Gain  Gain=A2_etm4_1
  Gain2 : Gain  Gain=A3_etm4_1
  Gain3 : Gain  Gain=A4_etm4_1
  Sum : Sum  Inputs=++++
  Transport Delay : TransportDelay  DelayTime=t1_etm4_1
  Transport Delay1 : TransportDelay  DelayTime=t2_etm4_1
  Transport Delay2 : TransportDelay  DelayTime=t3_etm4_1
  Out1 : Outport
  wires:
  In1/1 -> Gain1/1, Gain3/1, Gain2/1, Gain/1
  Gain1/1 -> Transport Delay/1
  Transport Delay/1 -> Sum/2
  Sum/1 -> Out1/1
  Gain2/1 -> Transport Delay1/1
  Gain/1 -> Sum/1
  Transport Delay1/1 -> Sum/3
  Gain3/1 -> Transport Delay2/1
  Transport Delay2/1 -> Sum/4

== system Model_3_1/3_1_theta1 bang 0 n1=1; n2=1 2/ETM2/ETM4 ==
  In1 : Inport
  Gain : Gain  Gain=A1_etm4_2
  Gain1 : Gain  Gain=A2_etm4_2
  Gain2 : Gain  Gain=A3_etm4_2
  Gain3 : Gain  Gain=A4_etm4_2
  Sum : Sum  Inputs=++++
  Transport Delay : TransportDelay  DelayTime=t1_etm4_2
  Transport Delay1 : TransportDelay  DelayTime=t2_etm4_2
  Transport Delay2 : TransportDelay  DelayTime=t3_etm4_2
  Out1 : Outport
  wires:
  In1/1 -> Gain1/1, Gain3/1, Gain2/1, Gain/1
  Gain1/1 -> Transport Delay/1
  Transport Delay/1 -> Sum/2
  Sum/1 -> Out1/1
  Gain2/1 -> Transport Delay1/1
  Gain/1 -> Sum/1
  Transport Delay1/1 -> Sum/3
  Gain3/1 -> Transport Delay2/1
  Transport Delay2/1 -> Sum/4

== system Model_3_1/3_1_theta1 bang 0 n1=1; n2=1 2/LT_2bo_1/Bo1_LT_1 ==
  Input : Inport  PortDimensions=2
      mask Display: e = 0.06;c1 = [120 230 180]/255;c2 = ([120 230 180]+0)/(256+128);c3 = ([120 230 180]+128)/(256+128);patch([0 1 1 0],[0 0 1 1],c1);patch([0 1 1 1-e 1-e 0+e],[0 0 1 1-e 0+e 0+e],c2);patch([0 0 1 1-e 0+e 0+e],[0 1 1 1-e 1-e 0+e],c3);plot([0 1 1 0 0],[0 0 1 1 0]);
  Layer 1 : Subsystem
      mask Display: e = 0.06;c1 = [120 150 230]/255;c2 = ([120 150 230]+0)/383;c3 = ([120 150 230]+128)/383;patch([0 1 1 0],[0 0 1 1],c1);patch([0 1 1 1-e 1-e 0+e],[0 0 1 1-e 0+e 0+e],c2);patch([0 0 1 1-e 0+e 0+e],[0 1 1 1-e 1-e 0+e],c3);plot([0 1 1 0 0],[0 0 1 1 0]);
  Layer 2 : Subsystem
      mask Display: e = 0.06;c1 = [120 150 230]/255;c2 = ([120 150 230]+0)/383;c3 = ([120 150 230]+128)/383;patch([0 1 1 0],[0 0 1 1],c1);patch([0 1 1 1-e 1-e 0+e],[0 0 1 1-e 0+e 0+e],c2);patch([0 0 1 1-e 0+e 0+e],[0 1 1 1-e 1-e 0+e],c3);plot([0 1 1 0 0],[0 0 1 1 0]);
  Process Input 1 : Subsystem
      mask Display: e = 0.06;c1 = [120 150 230]/255;c2 = ([120 150 230]+0)/383;c3 = ([120 150 230]+128)/383;patch([0 1 1 0],[0 0 1 1],c1);patch([0 1 1 1-e 1-e 0+e],[0 0 1 1-e 0+e 0+e],c2);patch([0 0 1 1-e 0+e 0+e],[0 1 1 1-e 1-e 0+e],c3);plot([0 1 1 0 0],[0 0 1 1 0]);
  Process Output 1 : Subsystem
      mask Display: e = 0.06;c1 = [120 150 230]/255;c2 = ([120 150 230]+0)/383;c3 = ([120 150 230]+128)/383;patch([0 1 1 0],[0 0 1 1],c1);patch([0 1 1 1-e 1-e 0+e],[0 0 1 1-e 0+e 0+e],c2);patch([0 0 1 1-e 0+e 0+e],[0 1 1 1-e 1-e 0+e],c3);plot([0 1 1 0 0],[0 0 1 1 0]);
  Output : Outport  InitialOutput=[0;0;0]
      mask Display: e = 0.06;c1 = [120 230 180]/255;c2 = ([120 230 180]+0)/(256+128);c3 = ([120 230 180]+128)/(256+128);patch([0 1 1 0],[0 0 1 1],c1);patch([0 1 1 1-e 1-e 0+e],[0 0 1 1-e 0+e 0+e],c2);patch([0 0 1 1-e 0+e 0+e],[0 1 1 1-e 1-e 0+e],c3);plot([0 1 1 0 0],[0 0 1 1 0]);
  wires:
  Input/1 -> Process Input 1/1(x)
  Process Output 1/1(y) -> Output/1
  Process Input 1/1(p) -> Layer 1/1("p{1}")
  Layer 1/1("a{1}") -> [feedback1]
  [feedback1] -> Layer 2/1("a{1} ")
  Layer 2/1("a{2}") -> Process Output 1/1(a)

== system Model_3_1/3_1_theta1 bang 0 n1=1; n2=1 2/LT_2bo_1/Bo2_LT_1 ==
  Input : Inport  PortDimensions=2
      mask Display: e = 0.06;c1 = [120 230 180]/255;c2 = ([120 230 180]+0)/(256+128);c3 = ([120 230 180]+128)/(256+128);patch([0 1 1 0],[0 0 1 1],c1);patch([0 1 1 1-e 1-e 0+e],[0 0 1 1-e 0+e 0+e],c2);patch([0 0 1 1-e 0+e 0+e],[0 1 1 1-e 1-e 0+e],c3);plot([0 1 1 0 0],[0 0 1 1 0]);
  Layer 1 : Subsystem
      mask Display: e = 0.06;c1 = [120 150 230]/255;c2 = ([120 150 230]+0)/383;c3 = ([120 150 230]+128)/383;patch([0 1 1 0],[0 0 1 1],c1);patch([0 1 1 1-e 1-e 0+e],[0 0 1 1-e 0+e 0+e],c2);patch([0 0 1 1-e 0+e 0+e],[0 1 1 1-e 1-e 0+e],c3);plot([0 1 1 0 0],[0 0 1 1 0]);
  Layer 2 : Subsystem
      mask Display: e = 0.06;c1 = [120 150 230]/255;c2 = ([120 150 230]+0)/383;c3 = ([120 150 230]+128)/383;patch([0 1 1 0],[0 0 1 1],c1);patch([0 1 1 1-e 1-e 0+e],[0 0 1 1-e 0+e 0+e],c2);patch([0 0 1 1-e 0+e 0+e],[0 1 1 1-e 1-e 0+e],c3);plot([0 1 1 0 0],[0 0 1 1 0]);
  Process Input 1 : Subsystem
      mask Display: e = 0.06;c1 = [120 150 230]/255;c2 = ([120 150 230]+0)/383;c3 = ([120 150 230]+128)/383;patch([0 1 1 0],[0 0 1 1],c1);patch([0 1 1 1-e 1-e 0+e],[0 0 1 1-e 0+e 0+e],c2);patch([0 0 1 1-e 0+e 0+e],[0 1 1 1-e 1-e 0+e],c3);plot([0 1 1 0 0],[0 0 1 1 0]);
  Process Output 1 : Subsystem
      mask Display: e = 0.06;c1 = [120 150 230]/255;c2 = ([120 150 230]+0)/383;c3 = ([120 150 230]+128)/383;patch([0 1 1 0],[0 0 1 1],c1);patch([0 1 1 1-e 1-e 0+e],[0 0 1 1-e 0+e 0+e],c2);patch([0 0 1 1-e 0+e 0+e],[0 1 1 1-e 1-e 0+e],c3);plot([0 1 1 0 0],[0 0 1 1 0]);
  Output : Outport  InitialOutput=[0;0;0]
      mask Display: e = 0.06;c1 = [120 230 180]/255;c2 = ([120 230 180]+0)/(256+128);c3 = ([120 230 180]+128)/(256+128);patch([0 1 1 0],[0 0 1 1],c1);patch([0 1 1 1-e 1-e 0+e],[0 0 1 1-e 0+e 0+e],c2);patch([0 0 1 1-e 0+e 0+e],[0 1 1 1-e 1-e 0+e],c3);plot([0 1 1 0 0],[0 0 1 1 0]);
  wires:
  Input/1 -> Process Input 1/1(x)
  Process Output 1/1(y) -> Output/1
  Process Input 1/1(p) -> Layer 1/1("p{1}")
  Layer 1/1("a{1}") -> [feedback1]
  [feedback1] -> Layer 2/1("a{1} ")
  Layer 2/1("a{2}") -> Process Output 1/1(a)

== system Model_3_1/3_1_theta1 bang 0 n1=1; n2=1 2/LT_2bo_1/PSO-ETM5 ==
  In1 : Inport
  Input : Inport  Port=2
  Input1 : Inport  Port=3
  Input2 : Inport  Port=4
  Gain : Gain  Gain=0.1667
  Gain1 : Gain  Gain=0.3333
  Gain2 : Gain  Gain=0.3333
  Gain3 : Gain  Gain=0.1667
  Sum : Sum  Inputs=++++
  Variable Transport Delay : VariableTransportDelay  VariableDelayType=Variable transport delay  MaximumDelay=10
  Variable Transport Delay1 : VariableTransportDelay  VariableDelayType=Variable transport delay  MaximumDelay=10
  Variable Transport Delay2 : VariableTransportDelay  VariableDelayType=Variable transport delay  MaximumDelay=10
  Out1 : Outport
  wires:
  In1/1 -> Gain1/1, Gain3/1, Gain2/1, Gain/1
  Gain1/1 -> Variable Transport Delay/1
  Variable Transport Delay/1 -> Sum/2
  Sum/1 -> Out1/1
  Gain2/1 -> Variable Transport Delay1/1
  Gain/1 -> Sum/1
  Variable Transport Delay1/1 -> Sum/3
  Gain3/1 -> Variable Transport Delay2/1
  Variable Transport Delay2/1 -> Sum/4
  Input/1 -> Variable Transport Delay/2
  Input1/1 -> Variable Transport Delay1/2
  Input2/1 -> Variable Transport Delay2/2

== system Model_3_1/3_1_theta1 bang 0 n1=1; n2=1 2/LT_2bo_1/PSO-ETM6 ==
  In1 : Inport
  Input : Inport  Port=2
  Input1 : Inport  Port=3
  Input2 : Inport  Port=4
  Gain : Gain  Gain=0.1667
  Gain1 : Gain  Gain=0.3333
  Gain2 : Gain  Gain=0.3333
  Gain3 : Gain  Gain=0.1667
  Sum : Sum  Inputs=++++
  Variable Transport Delay : VariableTransportDelay  VariableDelayType=Variable transport delay  MaximumDelay=10
  Variable Transport Delay1 : VariableTransportDelay  VariableDelayType=Variable transport delay  MaximumDelay=10
  Variable Transport Delay2 : VariableTransportDelay  VariableDelayType=Variable transport delay  MaximumDelay=10
  ref : Outport
  wires:
  In1/1 -> Gain1/1, Gain3/1, Gain2/1, Gain/1
  Gain1/1 -> Variable Transport Delay/1
  Variable Transport Delay/1 -> Sum/2
  Sum/1 -> ref/1
  Gain2/1 -> Variable Transport Delay1/1
  Gain/1 -> Sum/1
  Variable Transport Delay1/1 -> Sum/3
  Gain3/1 -> Variable Transport Delay2/1
  Variable Transport Delay2/1 -> Sum/4
  Input/1 -> Variable Transport Delay/2
  Input1/1 -> Variable Transport Delay1/2
  Input2/1 -> Variable Transport Delay2/2

== system Model_3_1/3_1_theta1 bang 0 n1=1; n2=1 2/LT_2bo_2/Bo1_LT_1 ==
  Input : Inport  PortDimensions=2
      mask Display: e = 0.06;c1 = [120 230 180]/255;c2 = ([120 230 180]+0)/(256+128);c3 = ([120 230 180]+128)/(256+128);patch([0 1 1 0],[0 0 1 1],c1);patch([0 1 1 1-e 1-e 0+e],[0 0 1 1-e 0+e 0+e],c2);patch([0 0 1 1-e 0+e 0+e],[0 1 1 1-e 1-e 0+e],c3);plot([0 1 1 0 0],[0 0 1 1 0]);
  Layer 1 : Subsystem
      mask Display: e = 0.06;c1 = [120 150 230]/255;c2 = ([120 150 230]+0)/383;c3 = ([120 150 230]+128)/383;patch([0 1 1 0],[0 0 1 1],c1);patch([0 1 1 1-e 1-e 0+e],[0 0 1 1-e 0+e 0+e],c2);patch([0 0 1 1-e 0+e 0+e],[0 1 1 1-e 1-e 0+e],c3);plot([0 1 1 0 0],[0 0 1 1 0]);
  Layer 2 : Subsystem
      mask Display: e = 0.06;c1 = [120 150 230]/255;c2 = ([120 150 230]+0)/383;c3 = ([120 150 230]+128)/383;patch([0 1 1 0],[0 0 1 1],c1);patch([0 1 1 1-e 1-e 0+e],[0 0 1 1-e 0+e 0+e],c2);patch([0 0 1 1-e 0+e 0+e],[0 1 1 1-e 1-e 0+e],c3);plot([0 1 1 0 0],[0 0 1 1 0]);
  Process Input 1 : Subsystem
      mask Display: e = 0.06;c1 = [120 150 230]/255;c2 = ([120 150 230]+0)/383;c3 = ([120 150 230]+128)/383;patch([0 1 1 0],[0 0 1 1],c1);patch([0 1 1 1-e 1-e 0+e],[0 0 1 1-e 0+e 0+e],c2);patch([0 0 1 1-e 0+e 0+e],[0 1 1 1-e 1-e 0+e],c3);plot([0 1 1 0 0],[0 0 1 1 0]);
  Process Output 1 : Subsystem
      mask Display: e = 0.06;c1 = [120 150 230]/255;c2 = ([120 150 230]+0)/383;c3 = ([120 150 230]+128)/383;patch([0 1 1 0],[0 0 1 1],c1);patch([0 1 1 1-e 1-e 0+e],[0 0 1 1-e 0+e 0+e],c2);patch([0 0 1 1-e 0+e 0+e],[0 1 1 1-e 1-e 0+e],c3);plot([0 1 1 0 0],[0 0 1 1 0]);
  Output : Outport  InitialOutput=[0;0;0]
      mask Display: e = 0.06;c1 = [120 230 180]/255;c2 = ([120 230 180]+0)/(256+128);c3 = ([120 230 180]+128)/(256+128);patch([0 1 1 0],[0 0 1 1],c1);patch([0 1 1 1-e 1-e 0+e],[0 0 1 1-e 0+e 0+e],c2);patch([0 0 1 1-e 0+e 0+e],[0 1 1 1-e 1-e 0+e],c3);plot([0 1 1 0 0],[0 0 1 1 0]);
  wires:
  Input/1 -> Process Input 1/1(x)
  Process Output 1/1(y) -> Output/1
  Process Input 1/1(p) -> Layer 1/1("p{1}")
  Layer 1/1("a{1}") -> [feedback1]
  [feedback1] -> Layer 2/1("a{1} ")
  Layer 2/1("a{2}") -> Process Output 1/1(a)

== system Model_3_1/3_1_theta1 bang 0 n1=1; n2=1 2/LT_2bo_2/Bo2_LT_1 ==
  Input : Inport  PortDimensions=2
      mask Display: e = 0.06;c1 = [120 230 180]/255;c2 = ([120 230 180]+0)/(256+128);c3 = ([120 230 180]+128)/(256+128);patch([0 1 1 0],[0 0 1 1],c1);patch([0 1 1 1-e 1-e 0+e],[0 0 1 1-e 0+e 0+e],c2);patch([0 0 1 1-e 0+e 0+e],[0 1 1 1-e 1-e 0+e],c3);plot([0 1 1 0 0],[0 0 1 1 0]);
  Layer 1 : Subsystem
      mask Display: e = 0.06;c1 = [120 150 230]/255;c2 = ([120 150 230]+0)/383;c3 = ([120 150 230]+128)/383;patch([0 1 1 0],[0 0 1 1],c1);patch([0 1 1 1-e 1-e 0+e],[0 0 1 1-e 0+e 0+e],c2);patch([0 0 1 1-e 0+e 0+e],[0 1 1 1-e 1-e 0+e],c3);plot([0 1 1 0 0],[0 0 1 1 0]);
  Layer 2 : Subsystem
      mask Display: e = 0.06;c1 = [120 150 230]/255;c2 = ([120 150 230]+0)/383;c3 = ([120 150 230]+128)/383;patch([0 1 1 0],[0 0 1 1],c1);patch([0 1 1 1-e 1-e 0+e],[0 0 1 1-e 0+e 0+e],c2);patch([0 0 1 1-e 0+e 0+e],[0 1 1 1-e 1-e 0+e],c3);plot([0 1 1 0 0],[0 0 1 1 0]);
  Process Input 1 : Subsystem
      mask Display: e = 0.06;c1 = [120 150 230]/255;c2 = ([120 150 230]+0)/383;c3 = ([120 150 230]+128)/383;patch([0 1 1 0],[0 0 1 1],c1);patch([0 1 1 1-e 1-e 0+e],[0 0 1 1-e 0+e 0+e],c2);patch([0 0 1 1-e 0+e 0+e],[0 1 1 1-e 1-e 0+e],c3);plot([0 1 1 0 0],[0 0 1 1 0]);
  Process Output 1 : Subsystem
      mask Display: e = 0.06;c1 = [120 150 230]/255;c2 = ([120 150 230]+0)/383;c3 = ([120 150 230]+128)/383;patch([0 1 1 0],[0 0 1 1],c1);patch([0 1 1 1-e 1-e 0+e],[0 0 1 1-e 0+e 0+e],c2);patch([0 0 1 1-e 0+e 0+e],[0 1 1 1-e 1-e 0+e],c3);plot([0 1 1 0 0],[0 0 1 1 0]);
  Output : Outport  InitialOutput=[0;0;0]
      mask Display: e = 0.06;c1 = [120 230 180]/255;c2 = ([120 230 180]+0)/(256+128);c3 = ([120 230 180]+128)/(256+128);patch([0 1 1 0],[0 0 1 1],c1);patch([0 1 1 1-e 1-e 0+e],[0 0 1 1-e 0+e 0+e],c2);patch([0 0 1 1-e 0+e 0+e],[0 1 1 1-e 1-e 0+e],c3);plot([0 1 1 0 0],[0 0 1 1 0]);
  wires:
  Input/1 -> Process Input 1/1(x)
  Process Output 1/1(y) -> Output/1
  Process Input 1/1(p) -> Layer 1/1("p{1}")
  Layer 1/1("a{1}") -> [feedback1]
  [feedback1] -> Layer 2/1("a{1} ")
  Layer 2/1("a{2}") -> Process Output 1/1(a)

== system Model_3_1/3_1_theta1 bang 0 n1=1; n2=1 2/LT_2bo_2/PSO-ETM5 ==
  In1 : Inport
  Input : Inport  Port=2
  Input1 : Inport  Port=3
  Input2 : Inport  Port=4
  Gain : Gain  Gain=0.1667
  Gain1 : Gain  Gain=0.3333
  Gain2 : Gain  Gain=0.3333
  Gain3 : Gain  Gain=0.1667
  Sum : Sum  Inputs=++++
  Variable Transport Delay : VariableTransportDelay  VariableDelayType=Variable transport delay  MaximumDelay=10
  Variable Transport Delay1 : VariableTransportDelay  VariableDelayType=Variable transport delay  MaximumDelay=10
  Variable Transport Delay2 : VariableTransportDelay  VariableDelayType=Variable transport delay  MaximumDelay=10
  Out1 : Outport
  wires:
  In1/1 -> Gain1/1, Gain3/1, Gain2/1, Gain/1
  Gain1/1 -> Variable Transport Delay/1
  Variable Transport Delay/1 -> Sum/2
  Sum/1 -> Out1/1
  Gain2/1 -> Variable Transport Delay1/1
  Gain/1 -> Sum/1
  Variable Transport Delay1/1 -> Sum/3
  Gain3/1 -> Variable Transport Delay2/1
  Variable Transport Delay2/1 -> Sum/4
  Input/1 -> Variable Transport Delay/2
  Input1/1 -> Variable Transport Delay1/2
  Input2/1 -> Variable Transport Delay2/2

== system Model_3_1/3_1_theta1 bang 0 n1=1; n2=1 2/LT_2bo_2/PSO-ETM6 ==
  In1 : Inport
  Input : Inport  Port=2
  Input1 : Inport  Port=3
  Input2 : Inport  Port=4
  Gain : Gain  Gain=0.1667
  Gain1 : Gain  Gain=0.3333
  Gain2 : Gain  Gain=0.3333
  Gain3 : Gain  Gain=0.1667
  Sum : Sum  Inputs=++++
  Variable Transport Delay : VariableTransportDelay  VariableDelayType=Variable transport delay  MaximumDelay=10
  Variable Transport Delay1 : VariableTransportDelay  VariableDelayType=Variable transport delay  MaximumDelay=10
  Variable Transport Delay2 : VariableTransportDelay  VariableDelayType=Variable transport delay  MaximumDelay=10
  ref : Outport
  wires:
  In1/1 -> Gain1/1, Gain3/1, Gain2/1, Gain/1
  Gain1/1 -> Variable Transport Delay/1
  Variable Transport Delay/1 -> Sum/2
  Sum/1 -> ref/1
  Gain2/1 -> Variable Transport Delay1/1
  Gain/1 -> Sum/1
  Variable Transport Delay1/1 -> Sum/3
  Gain3/1 -> Variable Transport Delay2/1
  Variable Transport Delay2/1 -> Sum/4
  Input/1 -> Variable Transport Delay/2
  Input1/1 -> Variable Transport Delay1/2
  Input2/1 -> Variable Transport Delay2/2

== system Model_3_1/3_1_theta1 bang 0 n1=1; n2=1 2/LT_chi_bo1_1/Bo1_LT_1 ==
  Input : Inport  PortDimensions=2
      mask Display: e = 0.06;c1 = [120 230 180]/255;c2 = ([120 230 180]+0)/(256+128);c3 = ([120 230 180]+128)/(256+128);patch([0 1 1 0],[0 0 1 1],c1);patch([0 1 1 1-e 1-e 0+e],[0 0 1 1-e 0+e 0+e],c2);patch([0 0 1 1-e 0+e 0+e],[0 1 1 1-e 1-e 0+e],c3);plot([0 1 1 0 0],[0 0 1 1 0]);
  Layer 1 : Subsystem
      mask Display: e = 0.06;c1 = [120 150 230]/255;c2 = ([120 150 230]+0)/383;c3 = ([120 150 230]+128)/383;patch([0 1 1 0],[0 0 1 1],c1);patch([0 1 1 1-e 1-e 0+e],[0 0 1 1-e 0+e 0+e],c2);patch([0 0 1 1-e 0+e 0+e],[0 1 1 1-e 1-e 0+e],c3);plot([0 1 1 0 0],[0 0 1 1 0]);
  Layer 2 : Subsystem
      mask Display: e = 0.06;c1 = [120 150 230]/255;c2 = ([120 150 230]+0)/383;c3 = ([120 150 230]+128)/383;patch([0 1 1 0],[0 0 1 1],c1);patch([0 1 1 1-e 1-e 0+e],[0 0 1 1-e 0+e 0+e],c2);patch([0 0 1 1-e 0+e 0+e],[0 1 1 1-e 1-e 0+e],c3);plot([0 1 1 0 0],[0 0 1 1 0]);
  Process Input 1 : Subsystem
      mask Display: e = 0.06;c1 = [120 150 230]/255;c2 = ([120 150 230]+0)/383;c3 = ([120 150 230]+128)/383;patch([0 1 1 0],[0 0 1 1],c1);patch([0 1 1 1-e 1-e 0+e],[0 0 1 1-e 0+e 0+e],c2);patch([0 0 1 1-e 0+e 0+e],[0 1 1 1-e 1-e 0+e],c3);plot([0 1 1 0 0],[0 0 1 1 0]);
  Process Output 1 : Subsystem
      mask Display: e = 0.06;c1 = [120 150 230]/255;c2 = ([120 150 230]+0)/383;c3 = ([120 150 230]+128)/383;patch([0 1 1 0],[0 0 1 1],c1);patch([0 1 1 1-e 1-e 0+e],[0 0 1 1-e 0+e 0+e],c2);patch([0 0 1 1-e 0+e 0+e],[0 1 1 1-e 1-e 0+e],c3);plot([0 1 1 0 0],[0 0 1 1 0]);
  Output : Outport  InitialOutput=[0;0;0]
      mask Display: e = 0.06;c1 = [120 230 180]/255;c2 = ([120 230 180]+0)/(256+128);c3 = ([120 230 180]+128)/(256+128);patch([0 1 1 0],[0 0 1 1],c1);patch([0 1 1 1-e 1-e 0+e],[0 0 1 1-e 0+e 0+e],c2);patch([0 0 1 1-e 0+e 0+e],[0 1 1 1-e 1-e 0+e],c3);plot([0 1 1 0 0],[0 0 1 1 0]);
  wires:
  Input/1 -> Process Input 1/1(x)
  Process Output 1/1(y) -> Output/1
  Process Input 1/1(p) -> Layer 1/1("p{1}")
  Layer 1/1("a{1}") -> [feedback1]
  [feedback1] -> Layer 2/1("a{1} ")
  Layer 2/1("a{2}") -> Process Output 1/1(a)

== system Model_3_1/3_1_theta1 bang 0 n1=1; n2=1 2/LT_chi_bo1_1/PSO-ETM2 ==
  In1 : Inport
  Input : Inport  Port=2
  Input1 : Inport  Port=3
  Input2 : Inport  Port=4
  Gain : Gain  Gain=0.1667
  Gain1 : Gain  Gain=0.3333
  Gain2 : Gain  Gain=0.3333
  Gain3 : Gain  Gain=0.1667
  Sum : Sum  Inputs=++++
  Variable Transport Delay : VariableTransportDelay  VariableDelayType=Variable transport delay  MaximumDelay=10
  Variable Transport Delay1 : VariableTransportDelay  VariableDelayType=Variable transport delay  MaximumDelay=10
  Variable Transport Delay2 : VariableTransportDelay  VariableDelayType=Variable transport delay  MaximumDelay=10
  ref : Outport
  wires:
  In1/1 -> Gain1/1, Gain3/1, Gain2/1, Gain/1
  Gain1/1 -> Variable Transport Delay/1
  Variable Transport Delay/1 -> Sum/2
  Sum/1 -> ref/1
  Gain2/1 -> Variable Transport Delay1/1
  Gain/1 -> Sum/1
  Variable Transport Delay1/1 -> Sum/3
  Gain3/1 -> Variable Transport Delay2/1
  Variable Transport Delay2/1 -> Sum/4
  Input/1 -> Variable Transport Delay/2
  Input1/1 -> Variable Transport Delay1/2
  Input2/1 -> Variable Transport Delay2/2

== system Model_3_1/3_1_theta1 bang 0 n1=1; n2=1 2/LT_chi_bo1_2/Bo1_LT_1 ==
  Input : Inport  PortDimensions=2
      mask Display: e = 0.06;c1 = [120 230 180]/255;c2 = ([120 230 180]+0)/(256+128);c3 = ([120 230 180]+128)/(256+128);patch([0 1 1 0],[0 0 1 1],c1);patch([0 1 1 1-e 1-e 0+e],[0 0 1 1-e 0+e 0+e],c2);patch([0 0 1 1-e 0+e 0+e],[0 1 1 1-e 1-e 0+e],c3);plot([0 1 1 0 0],[0 0 1 1 0]);
  Layer 1 : Subsystem
      mask Display: e = 0.06;c1 = [120 150 230]/255;c2 = ([120 150 230]+0)/383;c3 = ([120 150 230]+128)/383;patch([0 1 1 0],[0 0 1 1],c1);patch([0 1 1 1-e 1-e 0+e],[0 0 1 1-e 0+e 0+e],c2);patch([0 0 1 1-e 0+e 0+e],[0 1 1 1-e 1-e 0+e],c3);plot([0 1 1 0 0],[0 0 1 1 0]);
  Layer 2 : Subsystem
      mask Display: e = 0.06;c1 = [120 150 230]/255;c2 = ([120 150 230]+0)/383;c3 = ([120 150 230]+128)/383;patch([0 1 1 0],[0 0 1 1],c1);patch([0 1 1 1-e 1-e 0+e],[0 0 1 1-e 0+e 0+e],c2);patch([0 0 1 1-e 0+e 0+e],[0 1 1 1-e 1-e 0+e],c3);plot([0 1 1 0 0],[0 0 1 1 0]);
  Process Input 1 : Subsystem
      mask Display: e = 0.06;c1 = [120 150 230]/255;c2 = ([120 150 230]+0)/383;c3 = ([120 150 230]+128)/383;patch([0 1 1 0],[0 0 1 1],c1);patch([0 1 1 1-e 1-e 0+e],[0 0 1 1-e 0+e 0+e],c2);patch([0 0 1 1-e 0+e 0+e],[0 1 1 1-e 1-e 0+e],c3);plot([0 1 1 0 0],[0 0 1 1 0]);
  Process Output 1 : Subsystem
      mask Display: e = 0.06;c1 = [120 150 230]/255;c2 = ([120 150 230]+0)/383;c3 = ([120 150 230]+128)/383;patch([0 1 1 0],[0 0 1 1],c1);patch([0 1 1 1-e 1-e 0+e],[0 0 1 1-e 0+e 0+e],c2);patch([0 0 1 1-e 0+e 0+e],[0 1 1 1-e 1-e 0+e],c3);plot([0 1 1 0 0],[0 0 1 1 0]);
  Output : Outport  InitialOutput=[0;0;0]
      mask Display: e = 0.06;c1 = [120 230 180]/255;c2 = ([120 230 180]+0)/(256+128);c3 = ([120 230 180]+128)/(256+128);patch([0 1 1 0],[0 0 1 1],c1);patch([0 1 1 1-e 1-e 0+e],[0 0 1 1-e 0+e 0+e],c2);patch([0 0 1 1-e 0+e 0+e],[0 1 1 1-e 1-e 0+e],c3);plot([0 1 1 0 0],[0 0 1 1 0]);
  wires:
  Input/1 -> Process Input 1/1(x)
  Process Output 1/1(y) -> Output/1
  Process Input 1/1(p) -> Layer 1/1("p{1}")
  Layer 1/1("a{1}") -> [feedback1]
  [feedback1] -> Layer 2/1("a{1} ")
  Layer 2/1("a{2}") -> Process Output 1/1(a)

== system Model_3_1/3_1_theta1 bang 0 n1=1; n2=1 2/LT_chi_bo1_2/PSO-ETM2 ==
  In1 : Inport
  Input : Inport  Port=2
  Input1 : Inport  Port=3
  Input2 : Inport  Port=4
  Gain : Gain  Gain=0.1667
  Gain1 : Gain  Gain=0.3333
  Gain2 : Gain  Gain=0.3333
  Gain3 : Gain  Gain=0.1667
  Sum : Sum  Inputs=++++
  Variable Transport Delay : VariableTransportDelay  VariableDelayType=Variable transport delay  MaximumDelay=10
  Variable Transport Delay1 : VariableTransportDelay  VariableDelayType=Variable transport delay  MaximumDelay=10
  Variable Transport Delay2 : VariableTransportDelay  VariableDelayType=Variable transport delay  MaximumDelay=10
  ref : Outport
  wires:
  In1/1 -> Gain1/1, Gain3/1, Gain2/1, Gain/1
  Gain1/1 -> Variable Transport Delay/1
  Variable Transport Delay/1 -> Sum/2
  Sum/1 -> ref/1
  Gain2/1 -> Variable Transport Delay1/1
  Gain/1 -> Sum/1
  Variable Transport Delay1/1 -> Sum/3
  Gain3/1 -> Variable Transport Delay2/1
  Variable Transport Delay2/1 -> Sum/4
  Input/1 -> Variable Transport Delay/2
  Input1/1 -> Variable Transport Delay1/2
  Input2/1 -> Variable Transport Delay2/2
